simulink model "SP_Dynamic_17Okt_ExergyFlow"  (R2019b)
settings: Solver=FixedStepAuto  StartTime=0.0  StopTime=0  FixedStep=1/3600  RelTol=1e-3
model workspace (MAT data in the model file):
  AD : Simulink.Parameter (value not decoded)
  AG : Simulink.Parameter (value not decoded)
  AH : Simulink.Parameter (value not decoded)
  AV : Simulink.Parameter (value not decoded)
  AVP : Simulink.Parameter (value not decoded)
  BCHL : Simulink.Parameter (value not decoded)
  BCHV : Simulink.Parameter (value not decoded)
  BD : Simulink.Parameter (value not decoded)
  BG : Simulink.Parameter (value not decoded)
  BH : Simulink.Parameter (value not decoded)
  BVP : Simulink.Parameter (value not decoded)
  CD : Simulink.Parameter (value not decoded)
  CG : Simulink.Parameter (value not decoded)
  CH : Simulink.Parameter (value not decoded)
  CVP : Simulink.Parameter (value not decoded)
  XMW : Simulink.Parameter (value not decoded)
symbols that are objects in the model workspace (value not decoded): AD, AG, AH, AV, AVP, BD, BG, BH, BVP, CD, CG, CH, CVP, XMW
undefined symbols (not defined in the file or in its folder): magnitude, SETPT, XMEAS, XMV
libraries: mylib x165, dspindex x17
(part 3 of 10)

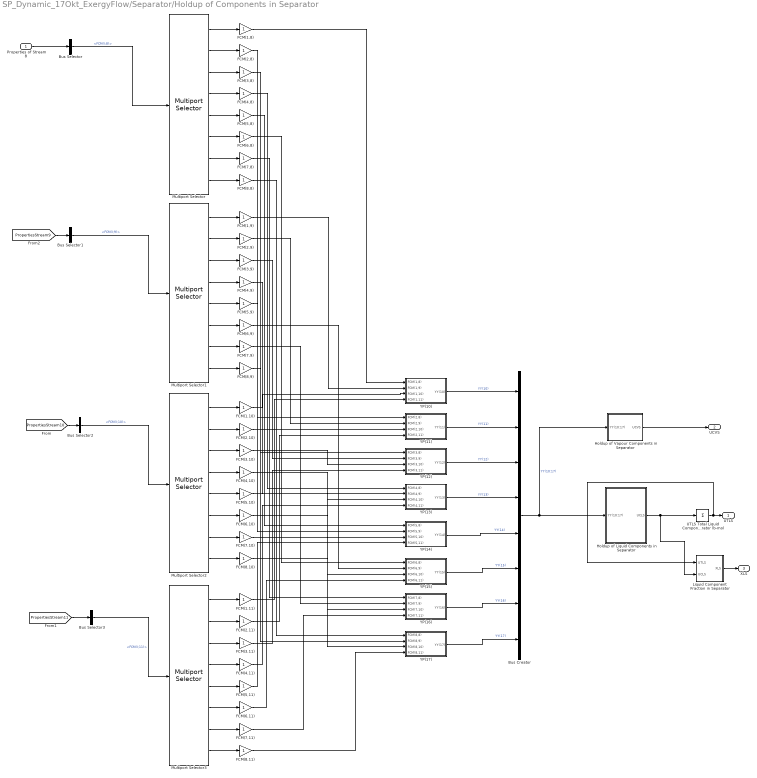
== system SP_Dynamic_17Okt_ExergyFlow/Separator/Holdup of Components in Separator ==
  Properties of Stream 8 : Inport
  Bus Creator : BusCreator  Inputs=8
  Bus Selector : BusSelector  OutputSignals=FCM(I;8)
  Bus Selector1 : BusSelector  OutputSignals=signal2.FCM(I;9)
  Bus Selector2 : BusSelector  OutputSignals=signal1.FCM(I;10)
  Bus Selector3 : BusSelector  OutputSignals=signal1.FCM(I;11)
  FCM(1,10) : Gain
  FCM(1,11) : Gain
  FCM(1,8) : Gain
  FCM(1,9) : Gain
  FCM(2,10) : Gain
  FCM(2,11) : Gain
  FCM(2,8) : Gain
  FCM(2,9) : Gain
  FCM(3,10) : Gain
  FCM(3,11) : Gain
  FCM(3,8) : Gain
  FCM(3,9) : Gain
  FCM(4,10) : Gain
  FCM(4,11) : Gain
  FCM(4,8) : Gain
  FCM(4,9) : Gain
  FCM(5,10) : Gain
  FCM(5,11) : Gain
  FCM(5,8) : Gain
  FCM(5,9) : Gain
  FCM(6,10) : Gain
  FCM(6,11) : Gain
  FCM(6,8) : Gain
  FCM(6,9) : Gain
  FCM(7,10) : Gain
  FCM(7,11) : Gain
  FCM(7,8) : Gain
  FCM(7,9) : Gain
  FCM(8,10) : Gain
  FCM(8,11) : Gain
  FCM(8,8) : Gain
  FCM(8,9) : Gain
  Holdup of Liquid Components in Separator : Subsystem
  Holdup of Vapour Components in Separator : Subsystem
  Liquid Component Fraction in Separator : Subsystem
  Multiport Selector : dspindex/Multiport Selector  rowsOrCols=Rows  idxCellArray={ 1,2,3,4,5,6,7,8}  idxErrMode=Clip Index
  Multiport Selector1 : dspindex/Multiport Selector  rowsOrCols=Rows  idxCellArray={ 1,2,3,4,5,6,7,8}  idxErrMode=Clip Index
  Multiport Selector2 : dspindex/Multiport Selector  rowsOrCols=Rows  idxCellArray={ 1,2,3,4,5,6,7,8}  idxErrMode=Clip Index
  Multiport Selector3 : dspindex/Multiport Selector  rowsOrCols=Rows  idxCellArray={1,2,3,4,5,6,7,8}  idxErrMode=Clip Index
  UTLS Total Liquid Component holdup in Separator lb-mol : Sum  Inputs=+
  YP(10) : Subsystem
  YP(11) : Subsystem
  YP(12) : Subsystem
  YP(13) : Subsystem
  YP(14) : Subsystem
  YP(15) : Subsystem
  YP(16) : Subsystem
  YP(17) : Subsystem
  UTLS : Outport  VectorParamsAs1DForOutWhenUnconnected=off
  UCVS : Outport  Port=2  VectorParamsAs1DForOutWhenUnconnected=off
  XLS : Outport  Port=3  VectorParamsAs1DForOutWhenUnconnected=off
  wires:
  Bus Selector/1 -> Multiport Selector/1  "<FCM(I;8)>"
  Multiport Selector/1 -> FCM(1,8)/1
  Multiport Selector/2 -> FCM(2,8)/1
  Multiport Selector/3 -> FCM(3,8)/1
  Multiport Selector/4 -> FCM(4,8)/1
  Multiport Selector/5 -> FCM(5,8)/1
  Multiport Selector/6 -> FCM(6,8)/1
  Multiport Selector/7 -> FCM(7,8)/1
  Multiport Selector/8 -> FCM(8,8)/1
  Multiport Selector1/1 -> FCM(1,9)/1
  Multiport Selector1/7 -> FCM(7,9)/1
  Multiport Selector1/2 -> FCM(2,9)/1
  Bus Selector1/1 -> Multiport Selector1/1  "<FCM(I;9)>"
  Multiport Selector1/3 -> FCM(3,9)/1
  Multiport Selector1/5 -> FCM(5,9)/1
  Multiport Selector1/4 -> FCM(4,9)/1
  Multiport Selector1/8 -> FCM(8,9)/1
  Multiport Selector1/6 -> FCM(6,9)/1
  FCM(1,8)/1 -> YP(10)/1(FCM(1,8))
  YP(10)/1(YY(10)) -> Bus Creator/1  "YY(10)"
  YP(11)/1(YY(11)) -> Bus Creator/2  "YY(11)"
  YP(12)/1(YY(12)) -> Bus Creator/3  "YY(12)"
  YP(13)/1("YY(13) ") -> Bus Creator/4  "YY(13)"
  YP(14)/1("YY(14) ") -> Bus Creator/5  "YY(14)"
  YP(15)/1("YY(15) ") -> Bus Creator/6  "YY(15)"
  YP(16)/1("YY(16) ") -> Bus Creator/7  "YY(16)"
  YP(17)/1("YY(17) ") -> Bus Creator/8  "YY(17)"
  Multiport Selector2/5 -> FCM(5,10)/1
  Multiport Selector2/7 -> FCM(7,10)/1
  Multiport Selector2/8 -> FCM(8,10)/1
  Multiport Selector2/3 -> FCM(3,10)/1
  Multiport Selector2/4 -> FCM(4,10)/1
  Bus Selector2/1 -> Multiport Selector2/1  "<FCM(I;10)>"
  Multiport Selector2/1 -> FCM(1,10)/1
  Multiport Selector2/2 -> FCM(2,10)/1
  Multiport Selector2/6 -> FCM(6,10)/1
  Multiport Selector3/5 -> FCM(5,11)/1
  Multiport Selector3/7 -> FCM(7,11)/1
  Multiport Selector3/8 -> FCM(8,11)/1
  Multiport Selector3/3 -> FCM(3,11)/1
  Multiport Selector3/4 -> FCM(4,11)/1
  Bus Selector3/1 -> Multiport Selector3/1  "<FCM(I;11)>"
  Multiport Selector3/1 -> FCM(1,11)/1
  Multiport Selector3/2 -> FCM(2,11)/1
  Multiport Selector3/6 -> FCM(6,11)/1
  FCM(1,9)/1 -> YP(10)/2(FCM(1,9))
  FCM(2,8)/1 -> YP(11)/1(FCM(2,8))
  FCM(3,8)/1 -> YP(12)/1(FCM(3,8))
  FCM(4,8)/1 -> YP(13)/1(FCM(4,8))
  FCM(5,8)/1 -> YP(14)/1(FCM(5,8))
  FCM(2,9)/1 -> YP(11)/2(FCM(2,9))
  FCM(3,9)/1 -> YP(12)/2(FCM(3,9))
  FCM(6,8)/1 -> YP(15)/1(FCM(6,8))
  FCM(7,8)/1 -> YP(16)/1(FCM(7,8))
  FCM(8,8)/1 -> YP(17)/1(FCM(8,8))
  FCM(4,9)/1 -> YP(13)/2(FCM(4,9))
  FCM(5,9)/1 -> YP(14)/2(FCM(5,9))
  FCM(6,9)/1 -> YP(15)/2(FCM(6,9))
  FCM(7,9)/1 -> YP(16)/2(FCM(7,9))
  FCM(8,9)/1 -> YP(17)/2(FCM(8,9))
  FCM(1,10)/1 -> YP(10)/3(FCM(1,10))
  FCM(2,10)/1 -> YP(11)/3(FCM(2,10))
  FCM(3,10)/1 -> YP(12)/3(FCM(3,10))
  FCM(4,10)/1 -> YP(13)/3(FCM(4,10))
  FCM(5,10)/1 -> YP(14)/3(FCM(5,10))
  FCM(6,10)/1 -> YP(15)/3(FCM(6,10))
  FCM(7,10)/1 -> YP(16)/3(FCM(7,10))
  FCM(8,10)/1 -> YP(17)/3(FCM(8,10))
  FCM(1,11)/1 -> YP(10)/4(FCM(1,11))
  FCM(2,11)/1 -> YP(11)/4(FCM(2,11))
  FCM(3,11)/1 -> YP(12)/4(FCM(3,11))
  FCM(4,11)/1 -> YP(13)/4(FCM(4,11))
  FCM(5,11)/1 -> YP(14)/4(FCM(5,11))
  FCM(6,11)/1 -> YP(15)/4(FCM(6,11))
  FCM(7,11)/1 -> YP(16)/4(FCM(7,11))
  FCM(8,11)/1 -> YP(17)/4(FCM(8,11))
  Holdup of Liquid Components in Separator/1(UCLS) -> UTLS Total Liquid Component holdup in Separator lb-mol/1, Liquid Component Fraction in Separator/2(UCLS)
  UTLS Total Liquid Component holdup in Separator lb-mol/1 -> UTLS/1, Liquid Component Fraction in Separator/1(UTLS)
  Bus Creator/1 -> Holdup of Vapour Components in Separator/1(YY(10:17)), Holdup of Liquid Components in Separator/1(YY(10:17))  "YY(10:17)"
  Holdup of Vapour Components in Separator/1(UCVS) -> UCVS/1
  Liquid Component Fraction in Separator/1(XLS) -> XLS/1
  Properties of Stream 8/1 -> Bus Selector/1
  [PropertiesStream9] -> Bus Selector1/1
  [PropertiesStream10] -> Bus Selector2/1
  [PropertiesStream11] -> Bus Selector3/1

== system SP_Dynamic_17Okt_ExergyFlow/Separator/Internal energy of separator ==
  Properties of Stream 8 : Inport
  Add : Sum  Inputs=+---+
  Bus Selector : BusSelector  OutputSignals=HST(8),FTM(8)
  Bus Selector1 : BusSelector  OutputSignals=signal2.HST(9),signal2.FTM(9)
  Bus Selector2 : BusSelector  OutputSignals=signal1.HST(10),signal1.FTM(10)
  Bus Selector3 : BusSelector  OutputSignals=signal1.HST(11),signal1.FTM(11)
  Product{,1..3} (4 alike) : Product
  YP(18) : Integrator  InitialConditionSource=external
  YY(18) : Constant  Value=0.5699317760
  "YY(18) " : Outport  VectorParamsAs1DForOutWhenUnconnected=off
  wires:
  Bus Selector/1 -> Product/1  "<HST(8)>"
  Bus Selector/2 -> Product/2  "<FTM(8)>"
  Bus Selector1/2 -> Product1/2  "<FTM(9)>"
  Bus Selector1/1 -> Product1/1  "<HST(9)>"
  Product/1 -> Add/1
  Product1/1 -> Add/2
  YP(18)/1 -> "YY(18) "/1
  YY(18)/1 -> YP(18)/2
  Add/1 -> YP(18)/1
  Bus Selector3/1 -> Product3/1  "<HST(11)>"
  Bus Selector2/2 -> Product2/2  "<FTM(10)>"
  Product2/1 -> Add/3
  Bus Selector3/2 -> Product3/2  "<FTM(11)>"
  Product3/1 -> Add/4
  Bus Selector2/1 -> Product2/1  "<HST(10)>"
  [QUS] -> Add/5
  Properties of Stream 8/1 -> Bus Selector/1
  [PropertiesStream9] -> Bus Selector1/1
  [PropertiesStream10] -> Bus Selector2/1
  [PropertiesStream11] -> Bus Selector3/1

== system SP_Dynamic_17Okt_ExergyFlow/Separator/Position of Valve 5 % ==
  Bus Selector : BusSelector  OutputSignals=XMV(5)
  Bus Selector1 : BusSelector  OutputSignals=IDV(19)
  Control valve : mylib/Control valve  SystemSampleTime=-1  Latency=0  AutoFrameSizeCalculation=off
  Divide : Product  Inputs=*/
  Subtract : Sum  Inputs=+-
  VTAU(5) : Constant  Value=7/3600
  YP(43) : Integrator  InitialConditionSource=external
  YY(43) : Constant  Value=22.21000000
  "YY(43) " : Outport  PortDimensions=1  VectorParamsAs1DForOutWhenUnconnected=off
  wires:
  Control valve/1 -> Subtract/1
  Subtract/1 -> Divide/1
  VTAU(5)/1 -> Divide/2
  Divide/1 -> YP(43)/1
  YP(43)/1 -> Subtract/2, "YY(43) "/1  "VPOS(5)"
  YY(43)/1 -> YP(43)/2
  [XMV] -> Bus Selector/1
  Bus Selector/1 -> Control valve/1  "<XMV(5)>"
  Bus Selector1/1 -> Control valve/2  "<IDV(19)>"
  [IDV] -> Bus Selector1/1

== system SP_Dynamic_17Okt_ExergyFlow/Separator/Position of Valve 6 % ==
  Bus Selector : BusSelector  OutputSignals=XMV(6)
  Control valve : mylib/Control valve  SystemSampleTime=-1  Latency=0  AutoFrameSizeCalculation=off
  Divide : Product  Inputs=*/
  IVST(6) : Constant  Value=0
  Subtract : Sum  Inputs=+-
  VTAU(6) : Constant  Value=5/3600
  YP(44) : Integrator  InitialConditionSource=external
  YY(44) : Constant  Value=40.06374673
  "YY(44) " : Outport  VectorParamsAs1DForOutWhenUnconnected=off
  wires:
  Control valve/1 -> Subtract/1
  Subtract/1 -> Divide/1
  VTAU(6)/1 -> Divide/2
  Divide/1 -> YP(44)/1
  YP(44)/1 -> "YY(44) "/1, Subtract/2  "VPOS(6)"
  YY(44)/1 -> YP(44)/2
  [XMV] -> Bus Selector/1
  Bus Selector/1 -> Control valve/1  "<XMV(6)>"
  IVST(6)/1 -> Control valve/2

== system SP_Dynamic_17Okt_ExergyFlow/Separator/Position of Valve 7 % ==
  Bus Selector : BusSelector  OutputSignals=XMV(7)
  Bus Selector1 : BusSelector  OutputSignals=IDV(19)
  Control valve : mylib/Control valve  SystemSampleTime=-1  Latency=0  AutoFrameSizeCalculation=off
  Divide : Product  Inputs=*/
  Subtract : Sum  Inputs=+-
  VTAU(7) : Constant  Value=5/3600
  YP(45) : Integrator  InitialConditionSource=external
  YY(45) : Constant  Value=38.10034370
  "YY(45) " : Outport  PortDimensions=1  VectorParamsAs1DForOutWhenUnconnected=off
  wires:
  Control valve/1 -> Subtract/1
  Subtract/1 -> Divide/1
  VTAU(7)/1 -> Divide/2
  Divide/1 -> YP(45)/1
  YP(45)/1 -> Subtract/2, "YY(45) "/1  "VPOS(7)"
  YY(45)/1 -> YP(45)/2
  [XMV] -> Bus Selector/1
  Bus Selector/1 -> Control valve/1  "<XMV(7)>"
  Bus Selector1/1 -> Control valve/2  "<IDV(19)>"
  [IDV] -> Bus Selector1/1

== system SP_Dynamic_17Okt_ExergyFlow/Separator/Pressure of Separator ==
  XLS : Inport  PortDimensions=8
  VVS : Inport  Port=2
  UCVS : Inport  Port=3
  Bus Creator1 : BusCreator  Inputs=8
  Demux : Demux  Outputs=5
  PPS(4) Partial pressure of Component D mmHg : Gain
  PPS(5) Partial pressure of Component E mmHg2 : Gain
  PPS(6) Partial pressure of Component F mmHg : Gain
  PPS(7) Partial pressure of Component H mmHg : Gain
  PPS(8) Partial pressure of Component G mmHg : Gain
  PPS(I) : Product
  PTS Total Pressure of Separator mmHg : Sum  Inputs=+
  Selector : Selector  InputPortWidth=8  IndexOptions=Index vector (dialog)  Indices=[4 5 6 7 8]  OutputSizes=1
  Selector1 : Selector  InputPortWidth=8  IndexOptions=Index vector (dialog)  Indices=[4 5 6 7 8]  OutputSizes=1
  Subsystem : Subsystem
  VPR Vapour Pressure mmHg : Subsystem
  PTS : Outport  PortDimensions=1  VectorParamsAs1DForOutWhenUnconnected=off
  PPS : Outport  Port=2  PortDimensions=8  VectorParamsAs1DForOutWhenUnconnected=off
  wires:
  PPS(8) Partial pressure of Component G mmHg/1 -> Bus Creator1/8  "PPS(8)"
  Bus Creator1/1 -> PPS/1, PTS Total Pressure of Separator mmHg/1
  PPS(7) Partial pressure of Component H mmHg/1 -> Bus Creator1/7  "PPS(7)"
  VPR Vapour Pressure mmHg/1(VPR) -> Selector1/1
  PPS(6) Partial pressure of Component F mmHg/1 -> Bus Creator1/6  "PPS(6)"
  Demux/2 -> PPS(5) Partial pressure of Component E mmHg2/1
  PTS Total Pressure of Separator mmHg/1 -> PTS/1
  Demux/1 -> PPS(4) Partial pressure of Component D mmHg/1
  Selector/1 -> PPS(I)/1
  PPS(5) Partial pressure of Component E mmHg2/1 -> Bus Creator1/5  "PPS(5)"
  PPS(I)/1 -> Demux/1
  Demux/5 -> PPS(8) Partial pressure of Component G mmHg/1
  Demux/4 -> PPS(7) Partial pressure of Component H mmHg/1
  PPS(4) Partial pressure of Component D mmHg/1 -> Bus Creator1/4  "PPS(4)"
  Selector1/1 -> PPS(I)/2
  Demux/3 -> PPS(6) Partial pressure of Component F mmHg/1
  [TCS] -> VPR Vapour Pressure mmHg/1(TCS), Subsystem/1(TCS)
  XLS/1 -> Selector/1
  VVS/1 -> Subsystem/2(VVS)
  UCVS/1 -> Subsystem/3(UCVS)
  Subsystem/1(PPS(1)) -> Bus Creator1/1  "PPS(1)"
  Subsystem/2(PPS(2)) -> Bus Creator1/2  "PPS(2)"
  Subsystem/3(PPS(3)) -> Bus Creator1/3  "PPS(3)"

== system SP_Dynamic_17Okt_ExergyFlow/Separator/Stream 10 ==
  XST(I,10) : Inport
  TST(10) : Inport  Port=2  PortDimensions=1
  VPOS(6) : Inport  Port=3  PortDimensions=1
  Bus Creator : BusCreator  Inputs=6
  FCM(I,10) Component molar flow of Stream 10 lb-mol/h : Product
  FTM(10) : Product  Inputs=*/
  HST(10) Molar Enthalpy of Stream 10 MBtu/lb-mol : Subsystem
  ITY : Constant
  Subsystem : Subsystem
  XMWS(10) Molecular weight of Stream 10 lb/lb-mol : Subsystem
  Properties of Stream 10 : Outport  VectorParamsAs1DForOutWhenUnconnected=off
  wires:
  XMWS(10) Molecular weight of Stream 10 lb/lb-mol/1(XMWS(10)) -> FTM(10)/2
  FTM(10)/1 -> Bus Creator/4, FCM(I,10) Component molar flow of Stream 10 lb-mol/h/2  "FTM(10)"
  ITY/1 -> Bus Creator/6, HST(10) Molar Enthalpy of Stream 10 MBtu/lb-mol/1(ITY)  "Phase"
  XST(I,10)/1 -> Bus Creator/1, FCM(I,10) Component molar flow of Stream 10 lb-mol/h/1, HST(10) Molar Enthalpy of Stream 10 MBtu/lb-mol/3(XST(I,I)), XMWS(10) Molecular weight of Stream 10 lb/lb-mol/1(XST(I,10))  "XST(I;10)"
  HST(10) Molar Enthalpy of Stream 10 MBtu/lb-mol/1("H ") -> Bus Creator/3  "HST(10)"
  TST(10)/1 -> Bus Creator/2, HST(10) Molar Enthalpy of Stream 10 MBtu/lb-mol/2(T)  "TST(10)"
  FCM(I,10) Component molar flow of Stream 10 lb-mol/h/1 -> Bus Creator/5  "FCM(I;10)"
  Bus Creator/1 -> Properties of Stream 10/1
  VPOS(6)/1 -> Subsystem/1(VPOS(6))
  Subsystem/1(Out1) -> FTM(10)/1

== system SP_Dynamic_17Okt_ExergyFlow/Separator/Stream 11 ==
  XST(I,11) : Inport  PortDimensions=8
  TST(11) : Inport  Port=2  PortDimensions=1
  VPOS(7) : Inport  Port=3
  "   " : Constant  Value=100
  Bus Creator : BusCreator  Inputs=6
  FCM(I,11) Component molar flow of Stream 11 lb-mol/h : Product
  FTM(11) : Product  Inputs=**/
  HST(10) Molar Enthalpy of Stream 10 MBtu/lb-mol : Subsystem
  ITY : Constant  Value=0
  VRNG(7) : Constant  Value=1500
  Properties of Stream 11 : Outport  VectorParamsAs1DForOutWhenUnconnected=off
  wires:
  FTM(11)/1 -> Bus Creator/4, FCM(I,11) Component molar flow of Stream 11 lb-mol/h/2  "FTM(11)"
  ITY/1 -> Bus Creator/6, HST(10) Molar Enthalpy of Stream 10 MBtu/lb-mol/1(ITY)  "Phase"
  XST(I,11)/1 -> FCM(I,11) Component molar flow of Stream 11 lb-mol/h/1, Bus Creator/1, HST(10) Molar Enthalpy of Stream 10 MBtu/lb-mol/3(XST(I,I))  "XST(I;11)"
  HST(10) Molar Enthalpy of Stream 10 MBtu/lb-mol/1("H ") -> Bus Creator/3  "HST(11)"
  TST(11)/1 -> Bus Creator/2, HST(10) Molar Enthalpy of Stream 10 MBtu/lb-mol/2(T)  "TST(11)"
  VPOS(7)/1 -> FTM(11)/1
  FCM(I,11) Component molar flow of Stream 11 lb-mol/h/1 -> Bus Creator/5  "FCM(I;11)"
  VRNG(7)/1 -> FTM(11)/2
  "   "/1 -> FTM(11)/3
  Bus Creator/1 -> Properties of Stream 11/1

== system SP_Dynamic_17Okt_ExergyFlow/Separator/Stream 9 ==
  TST(9) : Inport
  XTS(I,9) : Inport  Port=2
  VPOS(5) : Inport  Port=3
  "  " : Product  Inputs=*/
  Bus Creator : BusCreator  Inputs=7
  FCM(I,9) Component molar flow of Stream 9 lb-mol/h : Product
  FTM(9) : Product  Inputs=*/
  HST(9) Molar Enthalpy of Stream 9 MBtu/lb-mol : Subsystem
  "HST(9) " : Sum
  ITY : Constant
  Subsystem : Subsystem
  XMWS(9) Molecular weight of Stream 9 lb/lb-mol : Subsystem
  Properties of Stream 9 : Outport  VectorParamsAs1DForOutWhenUnconnected=off
  wires:
  XTS(I,9)/1 -> XMWS(9) Molecular weight of Stream 9 lb/lb-mol/1(XST(I,9)), FCM(I,9) Component molar flow of Stream 9 lb-mol/h/2, Bus Creator/1, HST(9) Molar Enthalpy of Stream 9 MBtu/lb-mol/3(XST(I,I))  "XST(I;9)"
  TST(9)/1 -> Bus Creator/2, HST(9) Molar Enthalpy of Stream 9 MBtu/lb-mol/2(T)  "TST(9)"
  XMWS(9) Molecular weight of Stream 9 lb/lb-mol/1(XMWS(9)) -> Bus Creator/6, FTM(9)/2  "XMWS(9)"
  FTM(9)/1 -> Bus Creator/4, "  "/2, FCM(I,9) Component molar flow of Stream 9 lb-mol/h/1  "FTM(9)"
  [CPDH] -> "  "/1
  HST(9) Molar Enthalpy of Stream 9 MBtu/lb-mol/1("H ") -> "HST(9) "/1
  "  "/1 -> "HST(9) "/2
  "HST(9) "/1 -> Bus Creator/3  "HST(9)"
  FCM(I,9) Component molar flow of Stream 9 lb-mol/h/1 -> Bus Creator/5  "FCM(I;9)"
  Bus Creator/1 -> Properties of Stream 9/1
  VPOS(5)/1 -> Subsystem/1(VPOS(5))
  Subsystem/1(Out1) -> FTM(9)/1
  ITY/1 -> Bus Creator/7, HST(9) Molar Enthalpy of Stream 9 MBtu/lb-mol/1(ITY)  "Phase"

== system SP_Dynamic_17Okt_ExergyFlow/Separator/TCS Initial Temperature in Separator °C  ==
  UTLS : Inport
  ETS : Inport  Port=2  PortDimensions=1
  XLS : Inport  Port=3  PortDimensions=8
  "AG(I) Coefficient A to determine Enthalpy MBtu/lb·°F " : Constant  Value=AG
  "AH(I) Coefficient A to determine Enthalpy MBtu/lb·°F " : Constant  Value=AH
  AV(I) Coefficient AV to determine Enthalpy MBtu/lb : Constant  Value=AV
  BG(I) Coefficient B to determine Enthalpy MBtu/lb·°F² : Constant  Value=BG
  BH(I) Coefficient B to determine Enthalpy MBtu/lb·°F² : Constant  Value=BH
  CG(I) Coefficient C to determine Enthalpy MBtu/lb·°F³ : Constant  Value=CG
  CH(I) Coefficient C to determine Enthalpy MBtu/lb·°F³ : Constant  Value=CH
  Delay : Delay  DelayLength=1  InitialCondition=0
  Display1 : Display
  Display4 : Display
  IC : InitialCondition  Value=0
  ITY : Constant  Value=0
  MATLAB Function : MATLAB Function  TreatAsAtomicUnit=on
  "XMW(I) Molecular weight of components lb/lb-mol " : Constant  Value=XMW
  TCS : Outport  PortDimensions=1  VectorParamsAs1DForOutWhenUnconnected=off
  wires:
  MATLAB Function/1(TCS) -> Delay/1, TCS/1, Display4/1
  IC/1 -> MATLAB Function/13("TCS ")
  "AG(I) Coefficient A to determine Enthalpy MBtu/lb·°F "/1 -> MATLAB Function/4(AG)
  AV(I) Coefficient AV to determine Enthalpy MBtu/lb/1 -> MATLAB Function/7(AV)
  MATLAB Function/2(J) -> Display1/1
  ETS/1 -> MATLAB Function/10(ETS)
  CH(I) Coefficient C to determine Enthalpy MBtu/lb·°F³/1 -> MATLAB Function/3(CH)
  UTLS/1 -> MATLAB Function/11(UTLS)
  ITY/1 -> MATLAB Function/12(ITY)
  "XMW(I) Molecular weight of components lb/lb-mol "/1 -> MATLAB Function/8(XMW)
  XLS/1 -> MATLAB Function/9(XLS)
  "AH(I) Coefficient A to determine Enthalpy MBtu/lb·°F "/1 -> MATLAB Function/1(AH)
  CG(I) Coefficient C to determine Enthalpy MBtu/lb·°F³/1 -> MATLAB Function/6(CG)
  BH(I) Coefficient B to determine Enthalpy MBtu/lb·°F²/1 -> MATLAB Function/2(BH)
  BG(I) Coefficient B to determine Enthalpy MBtu/lb·°F²/1 -> MATLAB Function/5(BG)
  Delay/1 -> IC/1

== system SP_Dynamic_17Okt_ExergyFlow/Separator/Total Vapour Component Holdup in Separator ==
  XVS : Inport
  VVS : Inport  Port=2
  Display9 : Display
  RG Universal Gas Constant ft³·mmHg/K·lb-mol : Constant  Value=998.9
  TKS Temperature in Separator K : Sum
  To Convert °C to K : Constant  Value=273.15
  "UCVS(I) Vapour Component Holdup in Separator lb-mol  " : Product  Inputs=**
  UTVS Total Vapour Component Holdup in Reactor lb-mol : Product  Inputs=**//
  wires:
  UTVS Total Vapour Component Holdup in Reactor lb-mol/1 -> "UCVS(I) Vapour Component Holdup in Separator lb-mol  "/1
  VVS/1 -> UTVS Total Vapour Component Holdup in Reactor lb-mol/2
  [PTS] -> UTVS Total Vapour Component Holdup in Reactor lb-mol/1
  XVS/1 -> "UCVS(I) Vapour Component Holdup in Separator lb-mol  "/2
  "UCVS(I) Vapour Component Holdup in Separator lb-mol  "/1 -> Display9/1
  RG Universal Gas Constant ft³·mmHg/K·lb-mol/1 -> UTVS Total Vapour Component Holdup in Reactor lb-mol/3
  TKS Temperature in Separator K/1 -> UTVS Total Vapour Component Holdup in Reactor lb-mol/4
  [TCS] -> TKS Temperature in Separator K/1
  To Convert °C to K/1 -> TKS Temperature in Separator K/2

== system SP_Dynamic_17Okt_ExergyFlow/Separator/Vapour Component Fraction in Separator ==
  PPS : Inport
  Bus Creator2 : BusCreator  Inputs=8
  Bus Selector1 : BusSelector  OutputSignals=PPS(1),PPS(2),PPS(3),PPS(4),PPS(5),PPS(6),PPS(7),PPS(8)
  XVS(1) : Product  Inputs=*/
  XVS(2) : Product  Inputs=*/
  XVS(3) : Product  Inputs=*/
  XVS(4) : Product  Inputs=*/
  XVS(5) : Product  Inputs=*/
  XVS(6) : Product  Inputs=*/
  XVS(7) : Product  Inputs=*/
  XVS(8) : Product  Inputs=*/
  XVS : Outport  PortDimensions=8  VectorParamsAs1DForOutWhenUnconnected=off
  wires:
  XVS(1)/1 -> Bus Creator2/1  "XVS(1)"
  Bus Selector1/5 -> XVS(5)/1  "<PPS(5)>"
  Bus Selector1/7 -> XVS(7)/1  "<PPS(7)>"
  Bus Selector1/6 -> XVS(6)/1  "<PPS(6)>"
  XVS(8)/1 -> Bus Creator2/8  "XVS(8)"
  Bus Selector1/8 -> XVS(8)/1  "<PPS(8)>"
  XVS(2)/1 -> Bus Creator2/2  "XVS(2)"
  [PTS] -> XVS(8)/2, XVS(7)/2, XVS(6)/2, XVS(5)/2, XVS(4)/2, XVS(3)/2, XVS(2)/2, XVS(1)/2
  Bus Selector1/2 -> XVS(2)/1  "<PPS(2)>"
  XVS(7)/1 -> Bus Creator2/7  "XVS(7)"
  Bus Selector1/4 -> XVS(4)/1  "<PPS(4)>"
  Bus Creator2/1 -> XVS/1
  XVS(4)/1 -> Bus Creator2/4  "XVS(4)"
  XVS(6)/1 -> Bus Creator2/6  "XVS(6)"
  Bus Selector1/3 -> XVS(3)/1  "<PPS(3)>"
  XVS(5)/1 -> Bus Creator2/5  "XVS(5)"
  PPS/1 -> Bus Selector1/1
  Bus Selector1/1 -> XVS(1)/1  "<PPS(1)>"
  XVS(3)/1 -> Bus Creator2/3  "XVS(3)"

== system SP_Dynamic_17Okt_ExergyFlow/Separator/Volume of Separator ==
  UTLS : Inport  PortDimensions=1
  XLS : Inport  Port=2  PortDimensions=8
  "DLS Molar Density of Liquids in Reactor lb-mol/ft³    " : Subsystem
  Display1 : Display
  "VLS Liquid Volume in Separator ft³ " : Product  Inputs=*/
  VTS Total Volume of Separator ft³ : Constant  Value=3500
  VVS Vapour Volume in Separator ft³ : Sum  Inputs=+-
  VVS : Outport  VectorParamsAs1DForOutWhenUnconnected=off
  VLS : Outport  Port=2  VectorParamsAs1DForOutWhenUnconnected=off
  tag scope: DLS=global
  wires:
  "VLS Liquid Volume in Separator ft³ "/1 -> VLS/1, VVS Vapour Volume in Separator ft³/2
  VVS Vapour Volume in Separator ft³/1 -> VVS/1
  UTLS/1 -> Display1/1, "VLS Liquid Volume in Separator ft³ "/1
  VTS Total Volume of Separator ft³/1 -> VVS Vapour Volume in Separator ft³/1
  "DLS Molar Density of Liquids in Reactor lb-mol/ft³    "/1("DLS ") -> [DLS], "VLS Liquid Volume in Separator ft³ "/2
  XLS/1 -> "DLS Molar Density of Liquids in Reactor lb-mol/ft³    "/1(XLS)
  [TCS] -> "DLS Molar Density of Liquids in Reactor lb-mol/ft³    "/2(TCS)

== system SP_Dynamic_17Okt_ExergyFlow/Shut Down Procedure/Reactor Level to High ==
  VLR : Inport
  Assertion : Assertion  AssertionFailFcn=|  StopWhenAssertionFail=off
      | set_param(bdroot,'SimulationCommand','stop'),
      | disp(sprintf('\nSimulation stoped.')), msgbox({'Plant Shutdown';'Reactor Level to High'}, 'Shutdown','error')
  Constant : Constant  Value=24
  Constant1 : Constant  Value=35.145
  Divide : Product  Inputs=*/
  Relational Operator : RelationalOperator  Operator=<  OutDataTypeStr=boolean  RndMeth=Simplest
  ISD : Outport  VectorParamsAs1DForOutWhenUnconnected=off
  wires:
  Relational Operator/1 -> ISD/1, Assertion/1
  Constant/1 -> Relational Operator/2
  Divide/1 -> Relational Operator/1
  VLR/1 -> Divide/1
  Constant1/1 -> Divide/2

== system SP_Dynamic_17Okt_ExergyFlow/Shut Down Procedure/Reactor Level to Low ==
  VLR : Inport
  Assertion : Assertion  AssertionFailFcn=|  StopWhenAssertionFail=off
      | set_param(bdroot,'SimulationCommand','stop'),
      | disp(sprintf('\nSimulation stoped.')), msgbox({'Plant Shutdown';'Reactor Level to Low'}, 'Shutdown','error')
  Constant : Constant  Value=2
  Constant1 : Constant  Value=35.145
  Divide : Product  Inputs=*/
  Relational Operator : RelationalOperator  Operator=>  OutDataTypeStr=boolean  RndMeth=Simplest
  ISD : Outport  VectorParamsAs1DForOutWhenUnconnected=off
  wires:
  Relational Operator/1 -> ISD/1, Assertion/1
  Constant/1 -> Relational Operator/2
  Divide/1 -> Relational Operator/1
  VLR/1 -> Divide/1
  Constant1/1 -> Divide/2

== system SP_Dynamic_17Okt_ExergyFlow/Shut Down Procedure/Reactor Presssure to High ==
  " " : Sum  Inputs=+-
  "    " : Constant  Value=760
  "       " : Constant  Value=101.325
  Assertion : Assertion  AssertionFailFcn=|  StopWhenAssertionFail=off
      | set_param(bdroot,'SimulationCommand','stop'),
      | disp(sprintf('\nSimulation stoped.')), msgbox({'Plant Shutdown';'Reactor Pressure to High'}, 'Shutdown','error')
  Constant : Constant  Value=3000
  Relational Operator : RelationalOperator  Operator=<  OutDataTypeStr=boolean  RndMeth=Simplest
  XMEAS(7) : Product  Inputs=*/*
  ISD : Outport  VectorParamsAs1DForOutWhenUnconnected=off
  wires:
  XMEAS(7)/1 -> Relational Operator/1
  Relational Operator/1 -> ISD/1, Assertion/1
  Constant/1 -> Relational Operator/2
  "       "/1 -> XMEAS(7)/3
  " "/1 -> XMEAS(7)/1
  [PTR] -> " "/1
  "    "/1 -> XMEAS(7)/2, " "/2

== system SP_Dynamic_17Okt_ExergyFlow/Shut Down Procedure/Reactor Temperature to High ==
  Assertion : Assertion  AssertionFailFcn=|  StopWhenAssertionFail=off
      | set_param(bdroot,'SimulationCommand','stop'),
      | disp(sprintf('\nSimulation stoped.')), msgbox({'Plant Shutdown';'Reactor Temperature to High'}, 'Shutdown','error')
  Constant : Constant  Value=175
  Relational Operator : RelationalOperator  Operator=<  OutDataTypeStr=boolean  RndMeth=Simplest
  ISD : Outport  VectorParamsAs1DForOutWhenUnconnected=off
  wires:
  [TCR] -> Relational Operator/1
  Relational Operator/1 -> ISD/1, Assertion/1
  Constant/1 -> Relational Operator/2

== system SP_Dynamic_17Okt_ExergyFlow/Shut Down Procedure/Separator Level to High ==
  VLS : Inport
  Assertion : Assertion  AssertionFailFcn=|  StopWhenAssertionFail=off
      | set_param(bdroot,'SimulationCommand','stop'),
      | disp(sprintf('\nSimulation stoped.')), msgbox({'Plant Shutdown';'Separator Level to High'}, 'Shutdown','error')
  Constant : Constant  Value=12
  Constant1 : Constant  Value=35.145
  Divide : Product  Inputs=*/
  Relational Operator : RelationalOperator  Operator=<  OutDataTypeStr=boolean  RndMeth=Simplest
  ISD : Outport  VectorParamsAs1DForOutWhenUnconnected=off
  wires:
  Relational Operator/1 -> ISD/1, Assertion/1
  Constant/1 -> Relational Operator/2
  Divide/1 -> Relational Operator/1
  VLS/1 -> Divide/1
  Constant1/1 -> Divide/2

== system SP_Dynamic_17Okt_ExergyFlow/Shut Down Procedure/Separator Level to Low ==
  VLS : Inport
  Assertion : Assertion  AssertionFailFcn=|  StopWhenAssertionFail=off
      | set_param(bdroot,'SimulationCommand','stop'),
      | disp(sprintf('\nSimulation stoped.')), msgbox({'Plant Shutdown';'Separator Level to Low'}, 'Shutdown','error')
  Constant : Constant
  Constant1 : Constant  Value=35.145
  Divide : Product  Inputs=*/
  Relational Operator : RelationalOperator  Operator=>  OutDataTypeStr=boolean  RndMeth=Simplest
  ISD : Outport  VectorParamsAs1DForOutWhenUnconnected=off
  wires:
  Relational Operator/1 -> ISD/1, Assertion/1
  Constant/1 -> Relational Operator/2
  Divide/1 -> Relational Operator/1
  VLS/1 -> Divide/1
  Constant1/1 -> Divide/2

== system SP_Dynamic_17Okt_ExergyFlow/Shut Down Procedure/Stripper Level to High ==
  VLC : Inport
  Assertion : Assertion  AssertionFailFcn=|  StopWhenAssertionFail=off
      | set_param(bdroot,'SimulationCommand','stop'),
      | disp(sprintf('\nSimulation stoped.')), msgbox({'Plant Shutdown';'Stripper Level to High'}, 'Shutdown','error')
  Constant : Constant  Value=8
  Constant1 : Constant  Value=35.145
  Display : Display
  Divide : Product  Inputs=*/
  Relational Operator : RelationalOperator  Operator=<  OutDataTypeStr=boolean  RndMeth=Simplest
  ISD : Outport  VectorParamsAs1DForOutWhenUnconnected=off
  wires:
  Relational Operator/1 -> ISD/1, Assertion/1
  Constant/1 -> Relational Operator/2
  VLC/1 -> Divide/1
  Constant1/1 -> Divide/2
  Divide/1 -> Display/1, Relational Operator/1

== system SP_Dynamic_17Okt_ExergyFlow/Shut Down Procedure/Stripper Level to Low ==
  VLC : Inport
  Assertion : Assertion  AssertionFailFcn=|  StopWhenAssertionFail=off
      | set_param(bdroot,'SimulationCommand','stop'),
      | disp(sprintf('\nSimulation stoped.')), msgbox({'Plant Shutdown';'Stripper Level to Low'}, 'Shutdown','error')
  Constant : Constant
  Constant1 : Constant  Value=35.145
  Divide : Product  Inputs=*/
  Relational Operator : RelationalOperator  Operator=>  OutDataTypeStr=boolean  RndMeth=Simplest
  ISD : Outport  VectorParamsAs1DForOutWhenUnconnected=off
  wires:
  Relational Operator/1 -> ISD/1, Assertion/1
  Constant/1 -> Relational Operator/2
  Divide/1 -> Relational Operator/1
  VLC/1 -> Divide/1
  Constant1/1 -> Divide/2

== system SP_Dynamic_17Okt_ExergyFlow/Stripper/Heat transfer of stripper ==
  VPOS(9) : Inport
  "  " : Constant  Value=0
  Add : Sum
  Bus Selector : BusSelector  OutputSignals=TESUB8(9)
  Constant : Constant
  Constant2 : Constant  Value=100
  If : If  IfExpression=u1 < 100
  If Action Subsystem : Subsystem  TreatAsAtomicUnit=on
  If Action Subsystem1 : Subsystem  TreatAsAtomicUnit=on
  Merge : Merge
  Product : Product
  Subtract : Sum  Inputs=+-
  UAC : Product  Inputs=***/
  VRNG(9) : Constant  Value=0.03
  tag scope: QUC=global
  wires:
  Constant/1 -> Add/1
  Bus Selector/1 -> Add/2  "<TESUB8(9)>"
  VPOS(9)/1 -> UAC/1
  VRNG(9)/1 -> UAC/2
  Add/1 -> UAC/3
  Constant2/1 -> Subtract/1, UAC/4
  If/1 -> If Action Subsystem/Action
  Product/1 -> If Action Subsystem/1(In1)
  [TCC] -> Subtract/2, If/1
  If/2 -> If Action Subsystem1/Action
  "  "/1 -> If Action Subsystem1/1(In1)
  Subtract/1 -> Product/2
  UAC/1 -> Product/1
  If Action Subsystem/1(Out1) -> Merge/1
  If Action Subsystem1/1(Out1) -> Merge/2
  Merge/1 -> [QUC]
  [TESUB8] -> Bus Selector/1

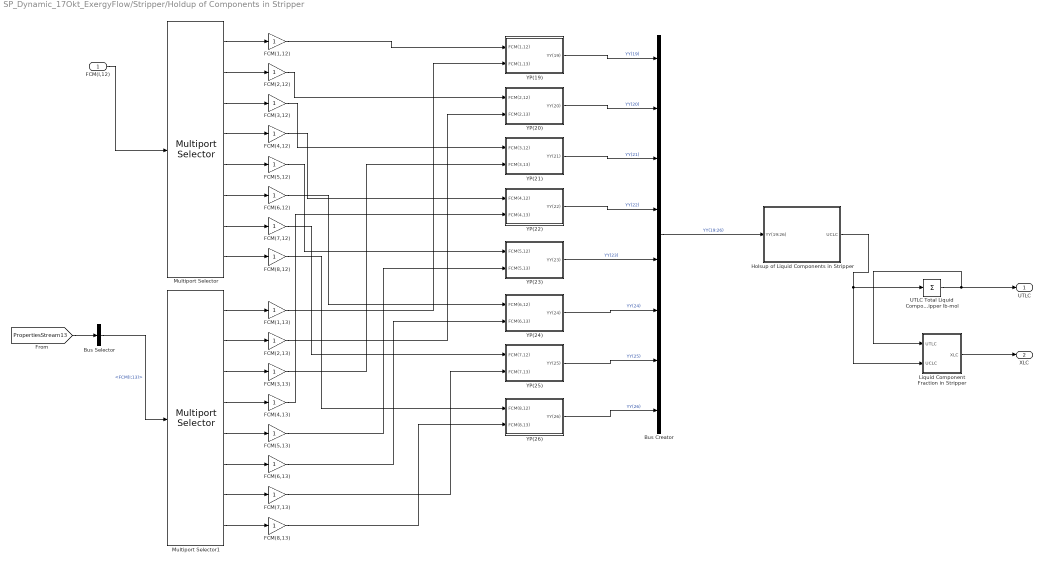
== system SP_Dynamic_17Okt_ExergyFlow/Stripper/Holdup of Components in Stripper ==
  "FCM(I,12) " : Inport
  Bus Creator : BusCreator  Inputs=8
  Bus Selector : BusSelector  OutputSignals=FCM(I;13)
  FCM(1,12) : Gain
  FCM(1,13) : Gain
  FCM(2,12) : Gain
  FCM(2,13) : Gain
  FCM(3,12) : Gain
  FCM(3,13) : Gain
  FCM(4,12) : Gain
  FCM(4,13) : Gain
  FCM(5,12) : Gain
  FCM(5,13) : Gain
  FCM(6,12) : Gain
  FCM(6,13) : Gain
  FCM(7,12) : Gain
  FCM(7,13) : Gain
  FCM(8,12) : Gain
  FCM(8,13) : Gain
  Holsup of Liquid Components in Stripper : Subsystem
  Liquid Component Fraction in Stripper : Subsystem
  Multiport Selector : dspindex/Multiport Selector  rowsOrCols=Rows  idxCellArray={ 1,2,3,4,5,6,7,8}  idxErrMode=Clip Index
  Multiport Selector1 : dspindex/Multiport Selector  rowsOrCols=Rows  idxCellArray={ 1,2,3,4,5,6,7,8}  idxErrMode=Clip Index
  UTLC Total Liquid Component holdup in Stripper lb-mol : Sum  Inputs=+
  YP(19) : Subsystem
  YP(20) : Subsystem
  YP(21) : Subsystem
  YP(22) : Subsystem
  YP(23) : Subsystem
  YP(24) : Subsystem
  YP(25) : Subsystem
  YP(26) : Subsystem
  UTLC : Outport  VectorParamsAs1DForOutWhenUnconnected=off
  XLC : Outport  Port=2  VectorParamsAs1DForOutWhenUnconnected=off
  wires:
  "FCM(I,12) "/1 -> Multiport Selector/1
  Multiport Selector/1 -> FCM(1,12)/1
  Multiport Selector/2 -> FCM(2,12)/1
  Multiport Selector/3 -> FCM(3,12)/1
  Multiport Selector/4 -> FCM(4,12)/1
  Multiport Selector/5 -> FCM(5,12)/1
  Multiport Selector/6 -> FCM(6,12)/1
  Multiport Selector/7 -> FCM(7,12)/1
  Multiport Selector/8 -> FCM(8,12)/1
  Multiport Selector1/1 -> FCM(1,13)/1
  Multiport Selector1/7 -> FCM(7,13)/1
  Multiport Selector1/2 -> FCM(2,13)/1
  Multiport Selector1/3 -> FCM(3,13)/1
  Multiport Selector1/5 -> FCM(5,13)/1
  Multiport Selector1/4 -> FCM(4,13)/1
  Multiport Selector1/8 -> FCM(8,13)/1
  Multiport Selector1/6 -> FCM(6,13)/1
  FCM(1,12)/1 -> YP(19)/1(FCM(1,12))
  YP(19)/1(YY(19)) -> Bus Creator/1  "YY(19)"
  YP(20)/1(YY(20)) -> Bus Creator/2  "YY(20)"
  YP(22)/1("YY(22)  ") -> Bus Creator/4  "YY(22)"
  YP(23)/1("YY(23)  ") -> Bus Creator/5  "YY(23)"
  YP(24)/1("YY(24)  ") -> Bus Creator/6  "YY(24)"
  YP(25)/1("YY(25)  ") -> Bus Creator/7  "YY(25)"
  YP(26)/1("YY(26)   ") -> Bus Creator/8  "YY(26)"
  FCM(1,13)/1 -> YP(19)/2(FCM(1,13))
  FCM(2,12)/1 -> YP(20)/1(FCM(2,12))
  FCM(3,12)/1 -> YP(21)/1(FCM(3,12))
  FCM(4,12)/1 -> YP(22)/1(FCM(4,12))
  FCM(5,12)/1 -> YP(23)/1(FCM(5,12))
  FCM(2,13)/1 -> YP(20)/2(FCM(2,13))
  FCM(3,13)/1 -> YP(21)/2(FCM(3,13))
  FCM(6,12)/1 -> YP(24)/1(FCM(6,12))
  FCM(7,12)/1 -> YP(25)/1(FCM(7,12))
  FCM(8,12)/1 -> YP(26)/1(FCM(8,12))
  FCM(4,13)/1 -> YP(22)/2(FCM(4,13))
  FCM(5,13)/1 -> YP(23)/2(FCM(5,13))
  FCM(6,13)/1 -> YP(24)/2(FCM(6,13))
  FCM(7,13)/1 -> YP(25)/2(FCM(7,13))
  FCM(8,13)/1 -> YP(26)/2(FCM(8,13))
  Bus Creator/1 -> Holsup of Liquid Components in Stripper/1(YY(19:26))  "YY(19:26)"
  Holsup of Liquid Components in Stripper/1(UCLC) -> Liquid Component Fraction in Stripper/2(UCLC), UTLC Total Liquid Component holdup in Stripper lb-mol/1
  YP(21)/1(YY(21)) -> Bus Creator/3  "YY(21)"
  UTLC Total Liquid Component holdup in Stripper lb-mol/1 -> Liquid Component Fraction in Stripper/1(UTLC), UTLC/1
  Liquid Component Fraction in Stripper/1(XLC) -> XLC/1
  [PropertiesStream13] -> Bus Selector/1
  Bus Selector/1 -> Multiport Selector1/1  "<FCM(I;13)>"

== system SP_Dynamic_17Okt_ExergyFlow/Stripper/Internal energy of stripper ==
  Properties of Stream 4 : Inport
  Properties of Stream 11 : Inport  Port=2
  Properties of Stream 5 : Inport  Port=3
  Add : Sum  Inputs=++--+
  Bus Selector : BusSelector  OutputSignals=HST(4),FTM(4)
  Bus Selector1 : BusSelector  OutputSignals=HST(11),FTM(11)
  Bus Selector2 : BusSelector  OutputSignals=HST(5),FTM(5)
  Bus Selector3 : BusSelector  OutputSignals=HST(13),FTM(13)
  Product{,1..3} (4 alike) : Product
  YP(27) : Integrator  InitialConditionSource=external
  YY(27) : Constant  Value=0.3755297257
  "YY(27) " : Outport  VectorParamsAs1DForOutWhenUnconnected=off
  wires:
  Bus Selector/1 -> Product/1  "<HST(4)>"
  Bus Selector/2 -> Product/2  "<FTM(4)>"
  Bus Selector1/2 -> Product1/2  "<FTM(11)>"
  Bus Selector1/1 -> Product1/1  "<HST(11)>"
  Product/1 -> Add/1
  Product1/1 -> Add/2
  YP(27)/1 -> "YY(27) "/1
  YY(27)/1 -> YP(27)/2
  Add/1 -> YP(27)/1
  Bus Selector3/1 -> Product3/1  "<HST(13)>"
  Bus Selector2/2 -> Product2/2  "<FTM(5)>"
  Product2/1 -> Add/3
  Bus Selector3/2 -> Product3/2  "<FTM(13)>"
  Product3/1 -> Add/4
  Bus Selector2/1 -> Product2/1  "<HST(5)>"
  [QUC] -> Add/5
  Properties of Stream 4/1 -> Bus Selector/1
  Properties of Stream 11/1 -> Bus Selector1/1
  Properties of Stream 5/1 -> Bus Selector2/1
  [PropertiesStream13] -> Bus Selector3/1

== system SP_Dynamic_17Okt_ExergyFlow/Stripper/PTC Pressure of Liquid zone in stripper mmHg ==
  UTLC : Inport
  TCC : Inport  Port=2
  PTC Total pressure of srtipper mmHg : Product  Inputs=***/
  RG Universal Gas Constant ft³·mmHg/K·lb-mol : Constant  Value=998.9
  TKC Temperature in Stripper K : Sum
  To Convert °C to K : Constant  Value=273.15
  tag scope: PTC=global
  wires:
  RG Universal Gas Constant ft³·mmHg/K·lb-mol/1 -> PTC Total pressure of srtipper mmHg/2
  [VLC] -> PTC Total pressure of srtipper mmHg/4
  TKC Temperature in Stripper K/1 -> PTC Total pressure of srtipper mmHg/3
  TCC/1 -> TKC Temperature in Stripper K/1
  PTC Total pressure of srtipper mmHg/1 -> [PTC]
  To Convert °C to K/1 -> TKC Temperature in Stripper K/2
  UTLC/1 -> PTC Total pressure of srtipper mmHg/1

== system SP_Dynamic_17Okt_ExergyFlow/Stripper/Position of Valve 8 % ==
  Bus Selector : BusSelector  OutputSignals=XMV(8)
  Bus Selector1 : BusSelector  OutputSignals=IDV(19)
  Control valve : mylib/Control valve  SystemSampleTime=-1  Latency=0  AutoFrameSizeCalculation=off
  Divide : Product  Inputs=*/
  Subtract : Sum  Inputs=+-
  VTAU(8) : Constant  Value=5/3600
  YP(46) : Integrator  InitialConditionSource=external
  YY(46) : Constant  Value=46.53415582
  "YY(46) " : Outport  PortDimensions=1  VectorParamsAs1DForOutWhenUnconnected=off
  wires:
  YP(46)/1 -> Subtract/2, "YY(46) "/1  "VPOS(8)"
  Subtract/1 -> Divide/1
  Control valve/1 -> Subtract/1
  VTAU(8)/1 -> Divide/2
  Divide/1 -> YP(46)/1
  YY(46)/1 -> YP(46)/2
  [XMV] -> Bus Selector/1
  Bus Selector/1 -> Control valve/1  "<XMV(8)>"
  [IDV] -> Bus Selector1/1
  Bus Selector1/1 -> Control valve/2  "<IDV(19)>"

== system SP_Dynamic_17Okt_ExergyFlow/Stripper/Position of Valve 9 % ==
  Bus Selector : BusSelector  OutputSignals=XMV(9)
  Bus Selector1 : BusSelector  OutputSignals=IDV(19)
  Control valve : mylib/Control valve  SystemSampleTime=-1  Latency=0  AutoFrameSizeCalculation=off
  Divide : Product  Inputs=*/
  Subtract : Sum  Inputs=+-
  VTAU(9) : Constant  Value=120/3600
  YP(47) : Integrator  InitialConditionSource=external
  YY(47) : Constant  Value=47.44573456
  "YY(47) " : Outport  PortDimensions=1  VectorParamsAs1DForOutWhenUnconnected=off
  wires:
  YP(47)/1 -> Subtract/2, "YY(47) "/1  "VPOS(9)"
  Subtract/1 -> Divide/1
  Control valve/1 -> Subtract/1
  VTAU(9)/1 -> Divide/2
  Divide/1 -> YP(47)/1
  YY(47)/1 -> YP(47)/2
  [XMV] -> Bus Selector/1
  Bus Selector/1 -> Control valve/1  "<XMV(9)>"
  Bus Selector1/1 -> Control valve/2  "<IDV(19)>"
  [IDV] -> Bus Selector1/1

== system SP_Dynamic_17Okt_ExergyFlow/Stripper/Split Fractions ==
  Bus Creator1 : BusCreator  Inputs=4
  SFR(1) : Constant  Value=0.99500
  SFR(2) : Constant  Value=0.99100
  SFR(3) : Constant  Value=0.99000
  Split fraction : Subsystem
  SFR : Outport  VectorParamsAs1DForOutWhenUnconnected=off
  wires:
  SFR(1)/1 -> Bus Creator1/1
  SFR(2)/1 -> Bus Creator1/2
  SFR(3)/1 -> Bus Creator1/3
  Split fraction/1(SFR) -> Bus Creator1/4
  Bus Creator1/1 -> SFR/1

== system SP_Dynamic_17Okt_ExergyFlow/Stripper/Stream 12 ==
  FCM(I,12) : Inport
  Bus Creator : BusCreator  Inputs=5
  Display : Display
  FTM(12) : Sum  Inputs=+
  Gain : Gain
  HST(12) Molar Enthalpy of Stream 12 MBtu/lb-mol : Subsystem
  ITY : Constant  Value=0
  XST(I,12) : Product  Inputs=*/
  wires:
  FTM(12)/1 -> XST(I,12)/2, Bus Creator/4  "FTM(12)"
  FCM(I,12)/1 -> XST(I,12)/1, Bus Creator/5, FTM(12)/1  "FCM(I;12)"
  XST(I,12)/1 -> Bus Creator/1, HST(12) Molar Enthalpy of Stream 12 MBtu/lb-mol/3(XST(I,I))  "XST(I;12)"
  [TCC] -> Gain/1
  Gain/1 -> Bus Creator/2, HST(12) Molar Enthalpy of Stream 12 MBtu/lb-mol/2(T)  "TST(12)"
  ITY/1 -> HST(12) Molar Enthalpy of Stream 12 MBtu/lb-mol/1(ITY)
  HST(12) Molar Enthalpy of Stream 12 MBtu/lb-mol/1("H ") -> Bus Creator/3  "HST(12)"
  Bus Creator/1 -> Display/1

== system SP_Dynamic_17Okt_ExergyFlow/Stripper/Stream 13 ==
  XST(I,13) : Inport  PortDimensions=8
  TST(13) : Inport  Port=2
  VPOS(8) : Inport  Port=3
  "   " : Constant  Value=100
  Bus Creator : BusCreator  Inputs=7
  FCM(I,13) Component molar flow of Stream 13 lb-mol/h : Product
  FTM(13) : Product  Inputs=**/
  HST(13) Molar Enthalpy of Stream 13 MBtu/lb-mol : Subsystem
  ITY : Constant  Value=0
  VRNG(8) : Constant  Value=1000
  Properties of Stream 13 : Outport  VectorParamsAs1DForOutWhenUnconnected=off
  wires:
  FTM(13)/1 -> Bus Creator/4, FCM(I,13) Component molar flow of Stream 13 lb-mol/h/2  "FTM(13)"
  ITY/1 -> Bus Creator/6, HST(13) Molar Enthalpy of Stream 13 MBtu/lb-mol/1(ITY)  "Phase"
  XST(I,13)/1 -> Bus Creator/1, FCM(I,13) Component molar flow of Stream 13 lb-mol/h/1, HST(13) Molar Enthalpy of Stream 13 MBtu/lb-mol/3(XST(I,I))  "XST(I;13)"
  HST(13) Molar Enthalpy of Stream 13 MBtu/lb-mol/1("H ") -> Bus Creator/3  "HST(13)"
  TST(13)/1 -> Bus Creator/2, HST(13) Molar Enthalpy of Stream 13 MBtu/lb-mol/2(T)  "TST(13)"
  VPOS(8)/1 -> FTM(13)/1
  FCM(I,13) Component molar flow of Stream 13 lb-mol/h/1 -> Bus Creator/5  "FCM(I;13)"
  VRNG(8)/1 -> FTM(13)/2
  "   "/1 -> FTM(13)/3
  Bus Creator/1 -> Properties of Stream 13/1
  [PTC] -> Bus Creator/7  "PTC"

== system SP_Dynamic_17Okt_ExergyFlow/Stripper/Stream 5 ==
  FCM(I,5) : Inport
  Bus Creator : BusCreator  Inputs=7
  FTM(5) : Sum  Inputs=+
  HST(5) Molar Enthalpy of Stream 5 MBtu/lb-mol : Subsystem
  ITY : Constant
  "TST(5) " : Gain
  XST(I,5) : Product  Inputs=*/
  Properties of Stream 5 : Outport  VectorParamsAs1DForOutWhenUnconnected=off
  tag scope: PropertiesStream5=global
  wires:
  FTM(5)/1 -> Bus Creator/4, XST(I,5)/2  "FTM(5)"
  FCM(I,5)/1 -> XST(I,5)/1, Bus Creator/5, FTM(5)/1  "FCM(I;5)"
  XST(I,5)/1 -> Bus Creator/1, HST(5) Molar Enthalpy of Stream 5 MBtu/lb-mol/3(XST(I,5))  "XST(I;5)"
  [TCC] -> "TST(5) "/1
  "TST(5) "/1 -> Bus Creator/2, HST(5) Molar Enthalpy of Stream 5 MBtu/lb-mol/2(TST(5))  "TST(5)"
  ITY/1 -> Bus Creator/6, HST(5) Molar Enthalpy of Stream 5 MBtu/lb-mol/1(ITY)  "Phase"
  HST(5) Molar Enthalpy of Stream 5 MBtu/lb-mol/1("H ") -> Bus Creator/3  "HST(5)"
  Bus Creator/1 -> [PropertiesStream5], Properties of Stream 5/1
  [PTV] -> Bus Creator/7

== system SP_Dynamic_17Okt_ExergyFlow/Stripper/TCC Initial Temperature in Stripper °C  ==
  UTLC : Inport  PortDimensions=1
  ETC : Inport  Port=2  PortDimensions=1
  XLC : Inport  Port=3  PortDimensions=8
  "AG(I) Coefficient A to determine Enthalpy MBtu/lb·°F " : Constant  Value=[3.411e-6;0.3799e-6;0.2491e-6;0.3567e-6;0.3463e-6;0.393e-6;0.17e-6;0.15e-6]
  "AH(I) Coefficient A to determine Enthalpy MBtu/lb·°F " : Constant  Value=[1e-6;1e-6;1e-6;0.96e-6;0.573e-6;0.652e-6;0.515e-6;0.471e-6]
  AV(I) Coefficient AV to determine Enthalpy MBtu/lb : Constant  Value=[1e-6;1e-6;1e-6;86.7e-6;160e-6;160e-6;225e-6;209e-6]
  BG(I) Coefficient B to determine Enthalpy MBtu/lb·°F² : Constant  Value=[7.18e-10;1.08e-9;1.36e-11;8.51e-10;8.96e-10;1.02e-9;0;0]
  BH(I) Coefficient B to determine Enthalpy MBtu/lb·°F² : Constant  Value=[0;0;0;8.7e-9;2.41e-9;2.18e-9;5.65e-10;8.7e-10]
  CG(I) Coefficient C to determine Enthalpy MBtu/lb·°F³ : Constant  Value=[6e-13;-3.98e-13;-3.93e-14;-3.12e-13;-3.27e-13;-3.12e-13;0;0]
  CH(I) Coefficient C to determine Enthalpy MBtu/lb·°F³ : Constant  Value=[0;0;0;4.81e-11;1.82e-11;1.94e-11;3.82e-12;2.62e-12]
  Delay : Delay  DelayLength=1  InitialCondition=0
  Display1 : Display
  Display4 : Display
  IC : InitialCondition  Value=0
  ITY : Constant  Value=0
  MATLAB Function : MATLAB Function  TreatAsAtomicUnit=on
  "XMW(I) Molecular weight of components lb/lb-mol " : Constant  Value=[2;25.4;28;32;46;48;62;76]
  TCC : Outport  PortDimensions=1  VectorParamsAs1DForOutWhenUnconnected=off
  wires:
  MATLAB Function/1(TCC) -> Delay/1, TCC/1, Display4/1
  IC/1 -> MATLAB Function/13("TCC ")
  "AG(I) Coefficient A to determine Enthalpy MBtu/lb·°F "/1 -> MATLAB Function/4(AG)
  AV(I) Coefficient AV to determine Enthalpy MBtu/lb/1 -> MATLAB Function/7(AV)
  MATLAB Function/2(J) -> Display1/1
  ETC/1 -> MATLAB Function/10(ETC)
  CH(I) Coefficient C to determine Enthalpy MBtu/lb·°F³/1 -> MATLAB Function/3(CH)
  UTLC/1 -> MATLAB Function/11(UTLC)
  ITY/1 -> MATLAB Function/12(ITY)
  "XMW(I) Molecular weight of components lb/lb-mol "/1 -> MATLAB Function/8(XMW)
  XLC/1 -> MATLAB Function/9(XLC)
  "AH(I) Coefficient A to determine Enthalpy MBtu/lb·°F "/1 -> MATLAB Function/1(AH)
  CG(I) Coefficient C to determine Enthalpy MBtu/lb·°F³/1 -> MATLAB Function/6(CG)
  BH(I) Coefficient B to determine Enthalpy MBtu/lb·°F²/1 -> MATLAB Function/2(BH)
  BG(I) Coefficient B to determine Enthalpy MBtu/lb·°F²/1 -> MATLAB Function/5(BG)
  Delay/1 -> IC/1

== system SP_Dynamic_17Okt_ExergyFlow/Stripper/Volume of Stripper ==
  UTLC : Inport  PortDimensions=1
  XLC : Inport  Port=2  PortDimensions=8
  "DLC Molar Density of Liquids in Stripper lb-mol/ft³    " : Subsystem
  "VLC Liquid Volume in Stripper ft³ " : Product  Inputs=*/
  tag scope: DLC=global, VLC=global
  wires:
  "DLC Molar Density of Liquids in Stripper lb-mol/ft³    "/1("DLC ") -> [DLC], "VLC Liquid Volume in Stripper ft³ "/2
  XLC/1 -> "DLC Molar Density of Liquids in Stripper lb-mol/ft³    "/1(XLC)
  "VLC Liquid Volume in Stripper ft³ "/1 -> [VLC]
  [TCC] -> "DLC Molar Density of Liquids in Stripper lb-mol/ft³    "/2(TCC)
  UTLC/1 -> "VLC Liquid Volume in Stripper ft³ "/1
